simulink model "chap11_8sim"  (Simulink 7.7)
settings: Solver=ode45  SolverMode=SingleTasking  StartTime=0.0  StopTime=30  FixedStep=0.001  RelTol=1e-3
settings Model: Creator=ljk  LastModifiedBy=ljk  ExtModeTrigMode=oneshot  ExtModeArmWhenConnect=off
settings DataIOCC: LimitDataPoints=off  SignalLoggingName=sigsOut
settings OptimizationCC: BooleanDataType=off
settings DebuggingCC: SaveWithParameterizedLinksMsg=none  SignalResolutionControl=TryResolveAllWithWarning  SolverPrmCheckMsg=none  MultiTaskDSMMsg=warning  MultiTaskCondExecSysMsg=none  StrictBusMsg=None
settings HardwareCC: TargetUnknown=on
settings RTWCC: IncludeERTFirstTime=on
settings CodeAppCC: CustomSymbolStrType=$N$R$M_T

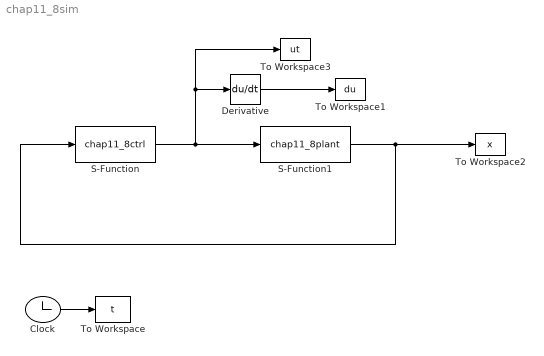
== system chap11_8sim ==
  Clock : Clock
  Derivative : Derivative
  S-Function : S-Function  FunctionName=chap11_8ctrl  EnableBusSupport=off
  S-Function1 : S-Function  FunctionName=chap11_8plant  EnableBusSupport=off
  To Workspace : ToWorkspace  VariableName=t  SampleTime=-1  SaveFormat=Array
  To Workspace1 : ToWorkspace  VariableName=du  SampleTime=-1  SaveFormat=Array
  To Workspace2 : ToWorkspace  VariableName=x  SampleTime=-1  SaveFormat=Array
  To Workspace3 : ToWorkspace  VariableName=ut  SampleTime=-1  SaveFormat=Array
  wires:
  Clock/1 -> To Workspace/1
  S-Function1/1 -> To Workspace2/1, S-Function/1
  S-Function/1 -> S-Function1/1, To Workspace3/1, Derivative/1
  Derivative/1 -> To Workspace1/1
